simulink model "untitled9"  (R2024a)
settings: Solver=VariableStepAuto  StartTime=0.0  StopTime=10.0  RelTol=1e-3
libraries: dspsrcs4 x2, dspfdesign x1
settings Model: Creator=LAPTOP  LastModifiedBy=LAPTOP

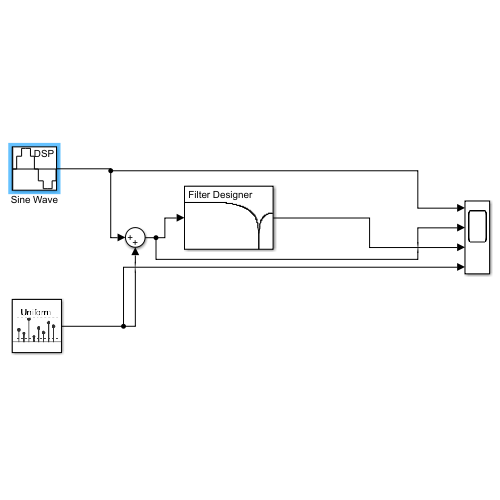
[thumbnail: Simulink's stored preview of the top-level diagram]
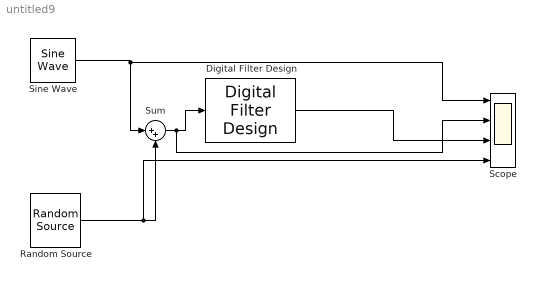
== system untitled9 ==
  Digital Filter Design : dspfdesign/Digital Filter Design  mwdsp_browser_bugfix_var=off
  Random Source : dspsrcs4/Random Source  SrcType=Uniform  MinVal=0  MaxVal=1  MeanVal=0  VarVal=1  RepMode=Specify seed  rawSeed=1  IsInherit=off  SampTime=1/1000  SampFrame=1  OutComplex=Real  DataType=double  SimulateUsing=Interpreted execution
  Scope : Scope  NumInputPorts=4
  Sine Wave : dspsrcs4/Sine Wave  Amplitude=1  Frequency=100  Phase=0  SampleMode=Discrete  OutComplex=Real  CompMethod=Trigonometric fcn  TableSize=Speed  SampleTime=1/1000  SamplesPerFrame=1  ResetState=Restart at time zero  OutputFrames=off  dataType=double  wordLen=16  udDataType=sfix(16)  fracBitsMode=Best precision  numFracBits=15  OutDataTypeStr=double  LastOutDataTypeStr=double
  Sum : Sum  Inputs=|++
  wires:
  Sine Wave/1 -> Scope/1, Sum/1
  Random Source/1 -> Scope/4, Sum/2
  Sum/1 -> Scope/2, Digital Filter Design/1
  Digital Filter Design/1 -> Scope/3
